simulink model "Main"  (R2025b)
settings: Solver=VariableStepAuto  StartTime=0.0  StopTime=20  RelTol=1e-3
PreLoadFcn:
  | Set_parameters
InitFcn:
  | Set_parameters;
values from neighbouring files (symbols this model uses):
  Date0 = 2460000    [Set_parameters.m]
undefined symbols (not defined in the file or in its folder): Aero, Init, Mass, Prop
libraries: simulink x1
settings Model: Creator=junho  LastModifiedBy=tmej1020

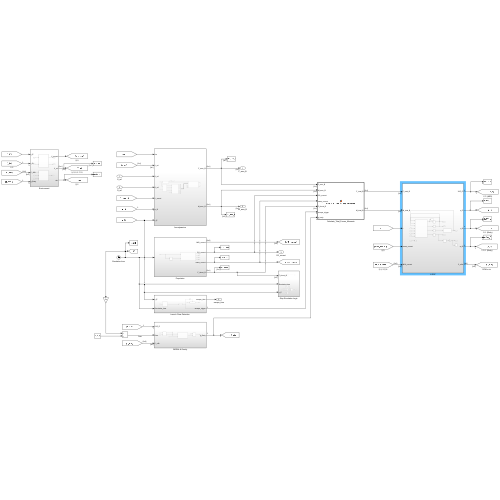
[thumbnail: Simulink's stored preview of the top-level diagram]
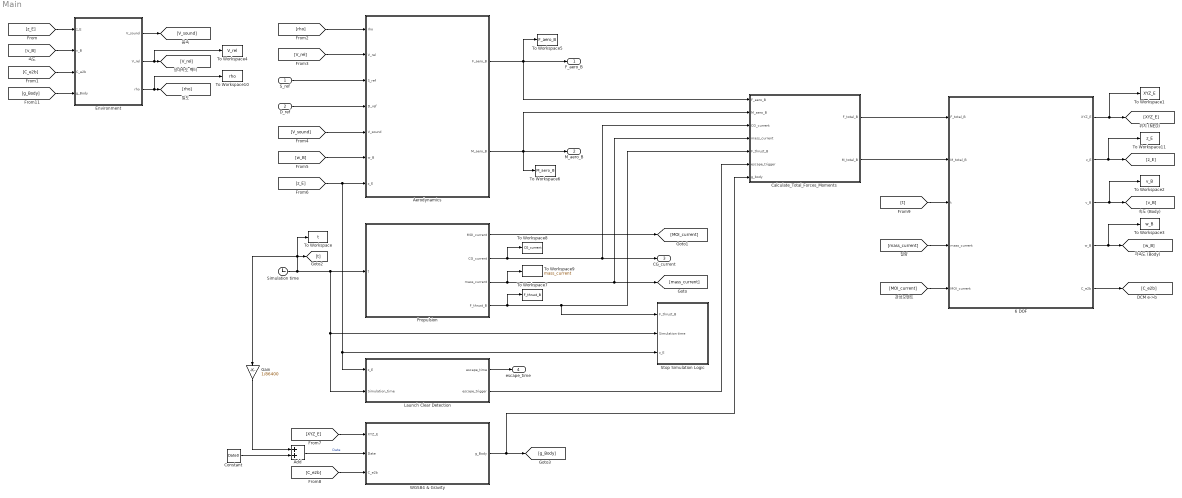
== system Main ==
  S_ref : Inport
  D_ref : Inport  Port=2
  "6 DOF " : Subsystem
  Add : Sum
  Aerodynamics : Subsystem
  Calculate_Total_Forces_Moments : MATLAB Function  TreatAsAtomicUnit=on
  Constant : Constant  Value=Date0
  Environment : Subsystem
  Gain : Gain  Gain=1/86400
  Launch Clear Detection : Subsystem
  Propulsion : Subsystem
  Simulation time : Clock
  Stop Simulation Logic : Subsystem
  To Workspace : ToWorkspace  VariableName=t  SampleTime=-1
  To Workspace1 : ToWorkspace  VariableName=XYZ_E  SampleTime=-1
  To Workspace10 : ToWorkspace  VariableName=rho  SaveFormat=Timeseries  SampleTime=-1
  To Workspace11 : ToWorkspace  VariableName=z_E  SampleTime=-1
  To Workspace2 : ToWorkspace  VariableName=v_B  SaveFormat=Timeseries  SampleTime=-1
  To Workspace3 : ToWorkspace  VariableName=w_B  SaveFormat=Timeseries  SampleTime=-1
  To Workspace4 : ToWorkspace  VariableName=V_rel  SaveFormat=Timeseries  SampleTime=-1
  To Workspace5 : ToWorkspace  VariableName=F_aero_B  SaveFormat=Timeseries  SampleTime=-1
  To Workspace6 : ToWorkspace  VariableName=M_aero_B  SaveFormat=Timeseries  SampleTime=-1
  To Workspace7 : ToWorkspace  VariableName=F_thrust_B  SampleTime=-1
  To Workspace8 : ToWorkspace  VariableName=CG_current  SaveFormat=Timeseries  SampleTime=-1
  To Workspace9 : ToWorkspace  VariableName=mass_current  SaveFormat=Timeseries  SampleTime=-1
  WGS84 & Gravity : Subsystem
  F_aero_B : Outport
  M_aero_B : Outport  Port=2
  CG_current : Outport  Port=3
  escape_time : Outport  Port=4
  wires:
  [XYZ_E] -> WGS84 & Gravity/1(XYZ_E)
  WGS84 & Gravity/1(g_Body) -> [g_Body], Calculate_Total_Forces_Moments/7(g_body)
  Add/1 -> WGS84 & Gravity/2(Date)  "Date"
  [C_e2b] -> WGS84 & Gravity/3(C_e2b)
  [rho] -> Aerodynamics/1(rho)
  [V_rel] -> Aerodynamics/2(V_rel)
  S_ref/1 -> Aerodynamics/3(S_ref)
  D_ref/1 -> Aerodynamics/4(D_ref)
  [V_sound] -> Aerodynamics/5(V_sound)
  [z_E] -> Launch Clear Detection/1(z_E), Stop Simulation Logic/3(z_E), Aerodynamics/7(z_E)
  Aerodynamics/1(F_aero_B) -> F_aero_B/1, Calculate_Total_Forces_Moments/1(F_aero_B), To Workspace5/1
  Aerodynamics/2(M_aero_B) -> M_aero_B/1, To Workspace6/1, Calculate_Total_Forces_Moments/2(M_aero_B)
  [w_B] -> Aerodynamics/6(w_B)
  Simulation time/1 -> Launch Clear Detection/2(Simulation_time), Stop Simulation Logic/2(Simulation time), Propulsion/1(t), To Workspace/1, Gain/1, [t]
  Propulsion/4(F_thrust_B) -> Stop Simulation Logic/1(F_thrust_B), Calculate_Total_Forces_Moments/5(F_thrust_B), To Workspace7/1
  Propulsion/1(MOI_current) -> [MOI_current]
  Propulsion/2(CG_current) -> To Workspace8/1, CG_current/1, Calculate_Total_Forces_Moments/3(CG_current)
  Propulsion/3(mass_current) -> To Workspace9/1, [mass_current], Calculate_Total_Forces_Moments/4(mass_current)
  Launch Clear Detection/1(escape_time) -> escape_time/1
  Launch Clear Detection/2(escape_trigger) -> Calculate_Total_Forces_Moments/6(escape_trigger)
  Calculate_Total_Forces_Moments/2(M_total_B) -> "6 DOF "/2(M_total_B)
  Calculate_Total_Forces_Moments/1(F_total_B) -> "6 DOF "/1(F_total_B)
  "6 DOF "/1(XYZ_E) -> [XYZ_E], To Workspace1/1
  [MOI_current] -> "6 DOF "/5(MOI_current)
  "6 DOF "/4(w_B) -> To Workspace3/1, [w_B]
  "6 DOF "/2(z_E) -> To Workspace11/1, [z_E]
  [mass_current] -> "6 DOF "/4(mass_current)
  "6 DOF "/3(v_B) -> To Workspace2/1, [v_B]
  "6 DOF "/5(C_e2b) -> [C_e2b]
  [v_B] -> Environment/2(v_B)
  Environment/3(rho) -> To Workspace10/1, [rho]
  [C_e2b] -> Environment/3(C_e2b)
  [z_E] -> Environment/1(z_E)
  Environment/2(V_rel) -> To Workspace4/1, [V_rel]
  Environment/1(V_sound) -> [V_sound]
  [t] -> "6 DOF "/3(t)
  Constant/1 -> Add/2
  Gain/1 -> Add/1
  [g_Body] -> Environment/4(g_Body)

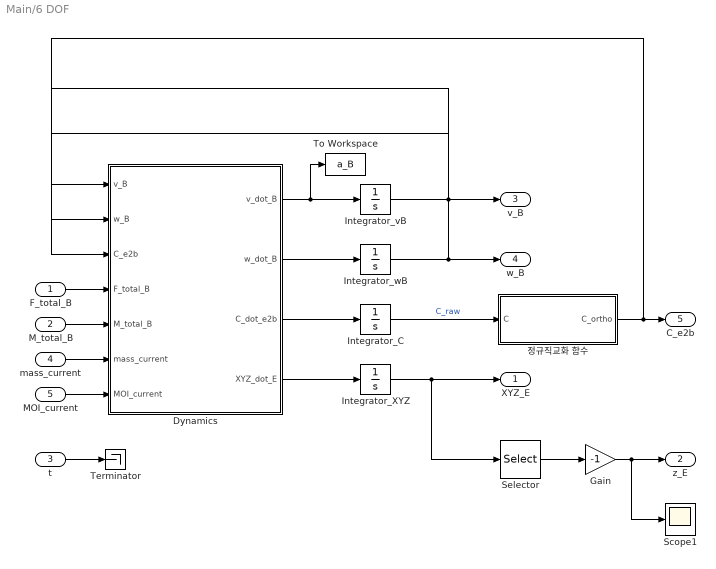
== system Main/6 DOF  ==
  F_total_B : Inport
  M_total_B : Inport  Port=2
  t : Inport  Port=3
  mass_current : Inport  Port=4
  MOI_current : Inport  Port=5
  Dynamics : MATLAB Function  TreatAsAtomicUnit=on
  Gain : Gain  Gain=-1
  Integrator_C : Integrator  InitialCondition=Init.C0_e2b
  Integrator_XYZ : Integrator  InitialCondition=zeros(3,1)
  Integrator_vB : Integrator  InitialCondition=zeros(3,1)
  Integrator_wB : Integrator  InitialCondition=zeros(3,1)
  Scope1 : Scope
      settings: ActiveDisplayYMinimum=-57.51768994793359  ActiveDisplayYMaximum=364.68499660349511
  Selector : Selector  InputPortWidth=3  IndexOptions=Index vector (dialog)  Indices=3  OutputSizes=1
  Terminator : Terminator
  To Workspace : ToWorkspace  VariableName=a_B  SaveFormat=Timeseries  SampleTime=-1
  정규직교화 함수 : MATLAB Function  TreatAsAtomicUnit=on
  XYZ_E : Outport
  z_E : Outport  Port=2
  v_B : Outport  Port=3
  w_B : Outport  Port=4
  C_e2b : Outport  Port=5
  wires:
  Integrator_vB/1 -> v_B/1, Dynamics/1(v_B)
  Integrator_wB/1 -> w_B/1, Dynamics/2(w_B)
  Integrator_XYZ/1 -> Selector/1, XYZ_E/1
  F_total_B/1 -> Dynamics/4(F_total_B)
  M_total_B/1 -> Dynamics/5(M_total_B)
  mass_current/1 -> Dynamics/6(mass_current)
  MOI_current/1 -> Dynamics/7(MOI_current)
  Dynamics/1(v_dot_B) -> To Workspace/1, Integrator_vB/1
  Dynamics/2(w_dot_B) -> Integrator_wB/1
  Dynamics/3(C_dot_e2b) -> Integrator_C/1
  Dynamics/4(XYZ_dot_E) -> Integrator_XYZ/1
  Selector/1 -> Gain/1
  Integrator_C/1 -> 정규직교화 함수/1(C)  "C_raw"
  정규직교화 함수/1(C_ortho) -> Dynamics/3(C_e2b), C_e2b/1
  t/1 -> Terminator/1
  Gain/1 -> Scope1/1, z_E/1

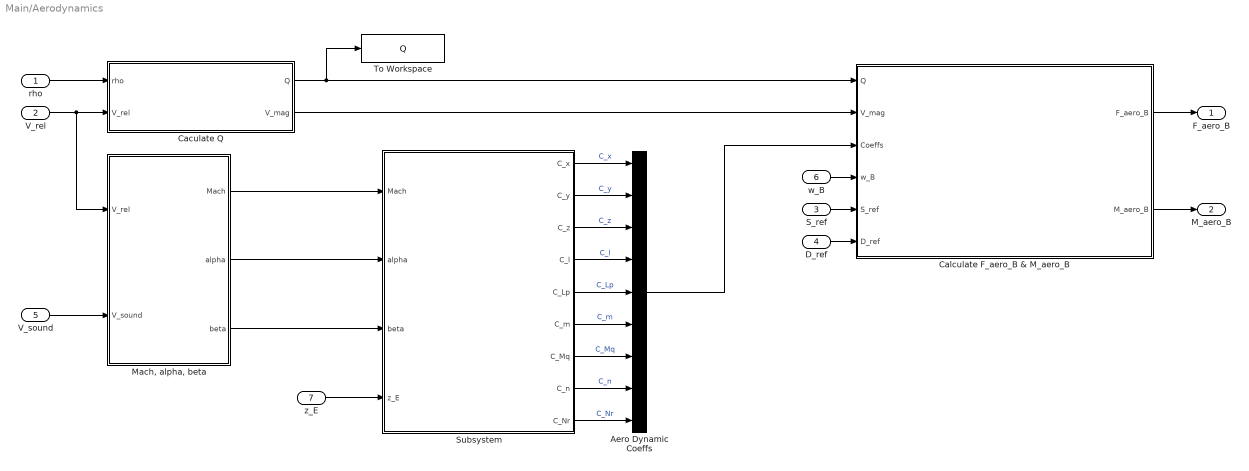
== system Main/Aerodynamics ==
  rho : Inport
  V_rel : Inport  Port=2
  S_ref : Inport  Port=3
  D_ref : Inport  Port=4
  V_sound : Inport  Port=5
  w_B : Inport  Port=6
  z_E : Inport  Port=7
  Aero Dynamic Coeffs : BusCreator  Inputs=9
  Caculate Q : MATLAB Function  TreatAsAtomicUnit=on
  Calculate F_aero_B & M_aero_B : MATLAB Function  TreatAsAtomicUnit=on
  "Mach, alpha, beta " : MATLAB Function  TreatAsAtomicUnit=on
  Subsystem : Subsystem
  To Workspace : ToWorkspace  VariableName=Q  SaveFormat=Timeseries  SampleTime=-1
  F_aero_B : Outport
  M_aero_B : Outport  Port=2
  wires:
  rho/1 -> Caculate Q/1(rho)
  V_rel/1 -> "Mach, alpha, beta "/1(V_rel), Caculate Q/2(V_rel)
  V_sound/1 -> "Mach, alpha, beta "/2(V_sound)
  "Mach, alpha, beta "/1(Mach) -> Subsystem/1(Mach)
  "Mach, alpha, beta "/2(alpha) -> Subsystem/2(alpha)
  "Mach, alpha, beta "/3(beta) -> Subsystem/3(beta)
  z_E/1 -> Subsystem/4(z_E)
  S_ref/1 -> Calculate F_aero_B & M_aero_B/5(S_ref)
  D_ref/1 -> Calculate F_aero_B & M_aero_B/6(D_ref)
  Aero Dynamic Coeffs/1 -> Calculate F_aero_B & M_aero_B/3(Coeffs)
  Calculate F_aero_B & M_aero_B/1(F_aero_B) -> F_aero_B/1
  Calculate F_aero_B & M_aero_B/2(M_aero_B) -> M_aero_B/1
  Subsystem/1(C_x) -> Aero Dynamic Coeffs/1  "C_x"
  Subsystem/2(C_y) -> Aero Dynamic Coeffs/2  "C_y"
  Subsystem/3(C_z) -> Aero Dynamic Coeffs/3  "C_z"
  Subsystem/4(C_l) -> Aero Dynamic Coeffs/4  "C_l"
  Subsystem/5(C_Lp) -> Aero Dynamic Coeffs/5  "C_Lp"
  Subsystem/6(C_m) -> Aero Dynamic Coeffs/6  "C_m"
  Subsystem/7(C_Mq) -> Aero Dynamic Coeffs/7  "C_Mq"
  Subsystem/8(C_n) -> Aero Dynamic Coeffs/8  "C_n"
  Subsystem/9(C_Nr) -> Aero Dynamic Coeffs/9  "C_Nr"
  Caculate Q/1(Q) -> To Workspace/1, Calculate F_aero_B & M_aero_B/1(Q)
  w_B/1 -> Calculate F_aero_B & M_aero_B/4(w_B)
  Caculate Q/2(V_mag) -> Calculate F_aero_B & M_aero_B/2(V_mag)

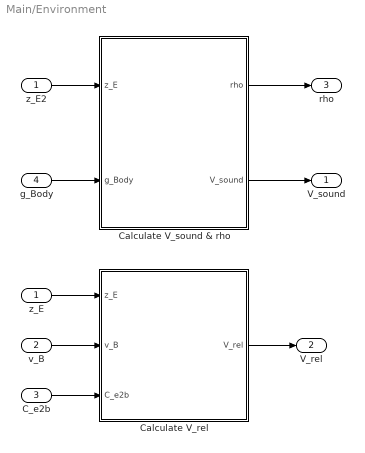
== system Main/Environment ==
  z_E : Inport
  v_B : Inport  Port=2
  C_e2b : Inport  Port=3
  g_Body : Inport  Port=4
  Calculate V_rel : MATLAB Function  TreatAsAtomicUnit=on
  Calculate V_sound & rho : MATLAB Function  TreatAsAtomicUnit=on
  z_E2 : InportShadow
  V_sound : Outport
  V_rel : Outport  Port=2
  rho : Outport  Port=3
  wires:
  z_E/1 -> Calculate V_rel/1(z_E)
  Calculate V_rel/1(V_rel) -> V_rel/1
  z_E2/1 -> Calculate V_sound & rho/1(z_E)
  Calculate V_sound & rho/2(V_sound) -> V_sound/1
  Calculate V_sound & rho/1(rho) -> rho/1
  v_B/1 -> Calculate V_rel/2(v_B)
  C_e2b/1 -> Calculate V_rel/3(C_e2b)
  g_Body/1 -> Calculate V_sound & rho/2(g_Body)

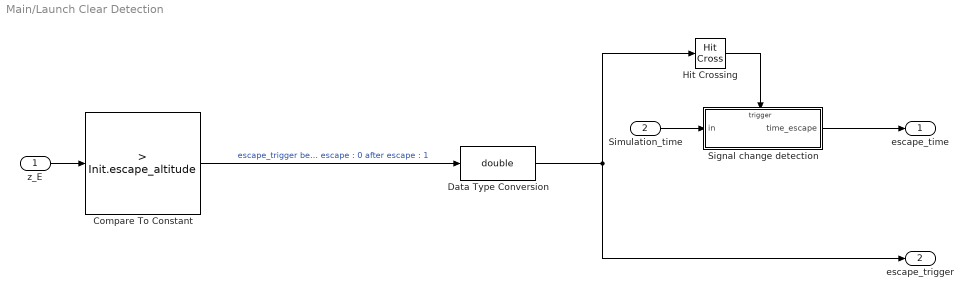
== system Main/Launch Clear Detection ==
  z_E : Inport
  Simulation_time : Inport  Port=2
  Compare To Constant : simulink/Logic and Bit Operations/Compare To Constant  relop=>  const=Init.escape_altitude  OutDataTypeStr=boolean
  Data Type Conversion : DataTypeConversion  OutDataTypeStr=double  SaturateOnIntegerOverflow=off  RndMeth=Floor
  Hit Crossing : HitCross  HitCrossingOffset=0.5  HitCrossingDirection=rising
  "Signal change detection " : Subsystem  TreatAsAtomicUnit=on
  escape_time : Outport
  escape_trigger : Outport  Port=2
  wires:
  z_E/1 -> Compare To Constant/1
  Compare To Constant/1 -> Data Type Conversion/1  "escape_trigger  before escape : 0 after escape : 1"
  Hit Crossing/1 -> "Signal change detection "/Trigger
  "Signal change detection "/1(time_escape) -> escape_time/1
  Data Type Conversion/1 -> escape_trigger/1, Hit Crossing/1
  Simulation_time/1 -> "Signal change detection "/1(in)

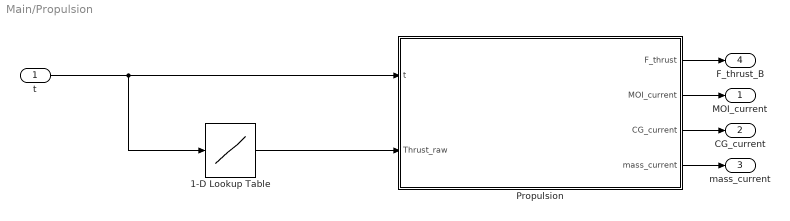
== system Main/Propulsion ==
  t : Inport
  1-D Lookup Table : Lookup_n-D  NumberOfTableDimensions=1  BreakpointsForDimension1=Prop.t_thrust  Table=Prop.F_thrust  ExtrapMethod=Clip  InternalRulePriority=Speed  RndMeth=Simplest
  Propulsion : MATLAB Function  TreatAsAtomicUnit=on
  MOI_current : Outport
  CG_current : Outport  Port=2
  mass_current : Outport  Port=3
  F_thrust_B : Outport  Port=4
  wires:
  t/1 -> 1-D Lookup Table/1, Propulsion/1(t)
  1-D Lookup Table/1 -> Propulsion/2(Thrust_raw)
  Propulsion/4(mass_current) -> mass_current/1
  Propulsion/3(CG_current) -> CG_current/1
  Propulsion/2(MOI_current) -> MOI_current/1
  Propulsion/1(F_thrust) -> F_thrust_B/1

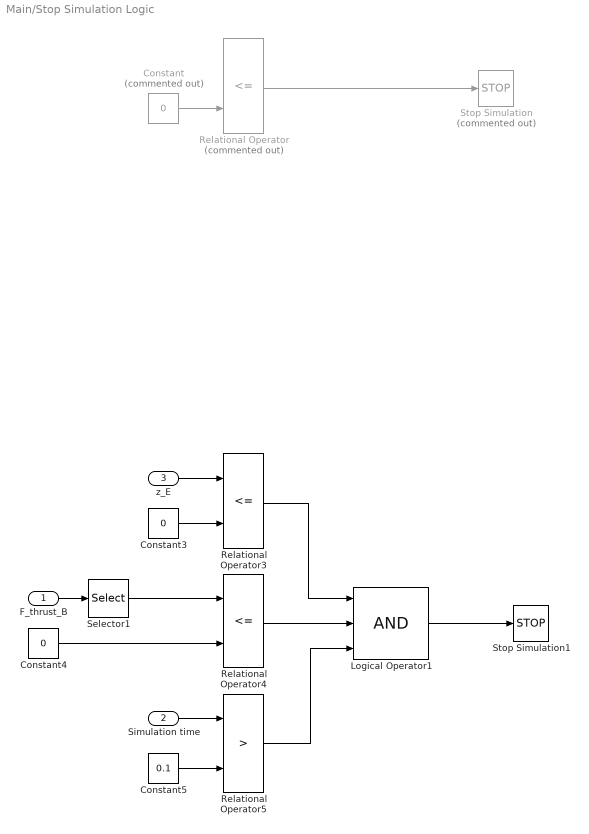
== system Main/Stop Simulation Logic ==
  F_thrust_B : Inport
  Simulation time : Inport  Port=2
  z_E : Inport  Port=3
  Constant : Constant  Commented=on  Value=0
  Constant3 : Constant  Value=0
  Constant4 : Constant  Value=0
  Constant5 : Constant  Value=0.1
  Logical Operator1 : Logic  Inputs=3  AllPortsSameDT=off  OutDataTypeStr=boolean
  Relational Operator : RelationalOperator  Commented=on  Operator=<=  OutDataTypeStr=boolean  RndMeth=Simplest  InputSameDT=off
  Relational Operator3 : RelationalOperator  Operator=<=  OutDataTypeStr=boolean  RndMeth=Simplest  InputSameDT=off
  Relational Operator4 : RelationalOperator  Operator=<=  OutDataTypeStr=boolean  RndMeth=Simplest  InputSameDT=off
  Relational Operator5 : RelationalOperator  Operator=>  OutDataTypeStr=boolean  RndMeth=Simplest  InputSameDT=off
  Selector1 : Selector  InputPortWidth=3  IndexOptions=Index vector (dialog)  Indices=1  OutputSizes=1
  Stop Simulation : Stop  Commented=on
  Stop Simulation1 : Stop
  wires:
  Relational Operator/1 -> Stop Simulation/1
  Constant/1 -> Relational Operator/2
  Selector1/1 -> Relational Operator4/1
  Relational Operator3/1 -> Logical Operator1/1
  Constant5/1 -> Relational Operator5/2
  Constant3/1 -> Relational Operator3/2
  Relational Operator5/1 -> Logical Operator1/3
  Constant4/1 -> Relational Operator4/2
  Relational Operator4/1 -> Logical Operator1/2
  Logical Operator1/1 -> Stop Simulation1/1
  z_E/1 -> Relational Operator3/1
  Simulation time/1 -> Relational Operator5/1
  F_thrust_B/1 -> Selector1/1

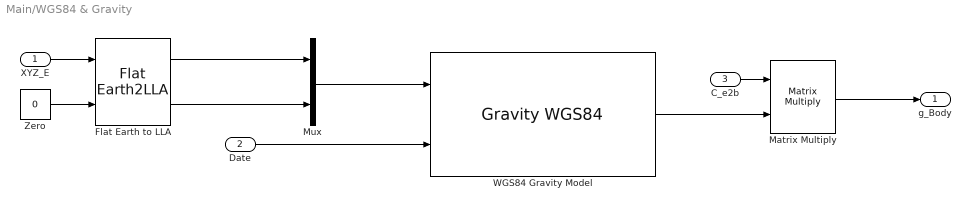
== system Main/WGS84 & Gravity ==
  XYZ_E : Inport
  Date : Inport  Port=2
  C_e2b : Inport  Port=3
  Flat Earth to LLA : FlatEarth2LLA  LL0=[Init.latitude_initial, Init.logitutde_initial]
  Matrix Multiply : Product  Multiplication=Matrix(*)
  Mux : Mux  Inputs=2
  "WGS84 Gravity Model  " : GravityWGS84  model=WGS84 Exact  no_atmos=off  jd_loc=on  month=February  day=19  year=2026  no_centrifugal=off
  Zero : Constant  Value=0  OutDataTypeStr=Inherit: Inherit via back propagation
  g_Body : Outport
  wires:
  XYZ_E/1 -> Flat Earth to LLA/1
  Date/1 -> "WGS84 Gravity Model  "/2
  Zero/1 -> Flat Earth to LLA/2
  Flat Earth to LLA/1 -> Mux/1
  Flat Earth to LLA/2 -> Mux/2
  Mux/1 -> "WGS84 Gravity Model  "/1
  "WGS84 Gravity Model  "/1 -> Matrix Multiply/2
  C_e2b/1 -> Matrix Multiply/1
  Matrix Multiply/1 -> g_Body/1

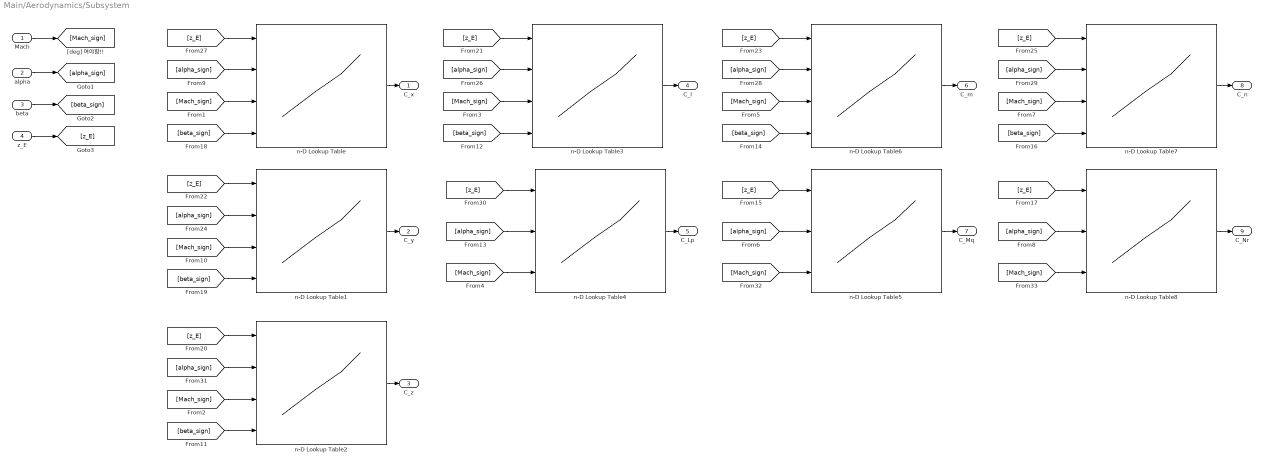
== system Main/Aerodynamics/Subsystem ==
  Mach : Inport
  alpha : Inport  Port=2
  beta : Inport  Port=3
  z_E : Inport  Port=4
  n-D Lookup Table : Lookup_n-D  NumberOfTableDimensions=4  BreakpointsForDimension1=Aero.altVec  BreakpointsForDimension2=Aero.alphaVec  BreakpointsForDimension3=Aero.machVec  BreakpointsForDimension4=Aero.betaVec  Table=Aero.CA_DB  InternalRulePriority=Speed  RndMeth=Simplest
      settings: InputPortMap=u0,u1,u2,u3
  n-D Lookup Table1 : Lookup_n-D  NumberOfTableDimensions=4  BreakpointsForDimension1=Aero.altVec  BreakpointsForDimension2=Aero.alphaVec  BreakpointsForDimension3=Aero.machVec  BreakpointsForDimension4=Aero.betaVec  Table=Aero.CY_DB  InternalRulePriority=Speed  RndMeth=Simplest
      settings: InputPortMap=u0,u1,u2,u3
  n-D Lookup Table2 : Lookup_n-D  NumberOfTableDimensions=4  BreakpointsForDimension1=Aero.altVec  BreakpointsForDimension2=Aero.alphaVec  BreakpointsForDimension3=Aero.machVec  BreakpointsForDimension4=Aero.betaVec  Table=Aero.CN_DB  InternalRulePriority=Speed  RndMeth=Simplest
      settings: InputPortMap=u0,u1,u2,u3
  n-D Lookup Table3 : Lookup_n-D  NumberOfTableDimensions=4  BreakpointsForDimension1=Aero.altVec  BreakpointsForDimension2=Aero.alphaVec  BreakpointsForDimension3=Aero.machVec  BreakpointsForDimension4=Aero.betaVec  Table=Aero.CLL_DB  InternalRulePriority=Speed  RndMeth=Simplest
      settings: InputPortMap=u0,u1,u2,u3
  n-D Lookup Table4 : Lookup_n-D  NumberOfTableDimensions=3  BreakpointsForDimension1=Aero.altVec_dynamic  BreakpointsForDimension2=Aero.alphaVec  BreakpointsForDimension3=Aero.machVec  Table=Aero.CLLP_DB  InternalRulePriority=Speed  RndMeth=Simplest
      settings: InputPortMap=u0,u1,u2
  n-D Lookup Table5 : Lookup_n-D  NumberOfTableDimensions=3  BreakpointsForDimension1=Aero.altVec_dynamic  BreakpointsForDimension2=Aero.alphaVec  BreakpointsForDimension3=Aero.machVec  Table=Aero.CMQ_DB  InternalRulePriority=Speed  RndMeth=Simplest
      settings: InputPortMap=u0,u1,u2
  n-D Lookup Table6 : Lookup_n-D  NumberOfTableDimensions=4  BreakpointsForDimension1=Aero.altVec  BreakpointsForDimension2=Aero.alphaVec  BreakpointsForDimension3=Aero.machVec  BreakpointsForDimension4=Aero.betaVec  Table=Aero.CM_DB  InternalRulePriority=Speed  RndMeth=Simplest
      settings: InputPortMap=u0,u1,u2,u3
  n-D Lookup Table7 : Lookup_n-D  NumberOfTableDimensions=4  BreakpointsForDimension1=Aero.altVec  BreakpointsForDimension2=Aero.alphaVec  BreakpointsForDimension3=Aero.machVec  BreakpointsForDimension4=Aero.betaVec  Table=Aero.CLN_DB  InternalRulePriority=Speed  RndMeth=Simplest
      settings: InputPortMap=u0,u1,u2,u3
  n-D Lookup Table8 : Lookup_n-D  NumberOfTableDimensions=3  BreakpointsForDimension1=Aero.altVec_dynamic  BreakpointsForDimension2=Aero.alphaVec  BreakpointsForDimension3=Aero.machVec  Table=Aero.CLNR_DB  InternalRulePriority=Speed  RndMeth=Simplest
      settings: InputPortMap=u0,u1,u2
  C_x : Outport
  C_y : Outport  Port=2
  C_z : Outport  Port=3
  C_l : Outport  Port=4
  C_Lp : Outport  Port=5
  C_m : Outport  Port=6
  C_Mq : Outport  Port=7
  C_n : Outport  Port=8
  C_Nr : Outport  Port=9
  wires:
  Mach/1 -> [Mach_sign]
  alpha/1 -> [alpha_sign]
  beta/1 -> [beta_sign]
  z_E/1 -> [z_E]
  n-D Lookup Table/1 -> C_x/1
  n-D Lookup Table1/1 -> C_y/1
  n-D Lookup Table2/1 -> C_z/1
  n-D Lookup Table3/1 -> C_l/1
  n-D Lookup Table4/1 -> C_Lp/1
  n-D Lookup Table6/1 -> C_m/1
  n-D Lookup Table5/1 -> C_Mq/1
  n-D Lookup Table7/1 -> C_n/1
  n-D Lookup Table8/1 -> C_Nr/1
  [alpha_sign] -> n-D Lookup Table4/2
  [z_E] -> n-D Lookup Table/1
  [alpha_sign] -> n-D Lookup Table/2
  [Mach_sign] -> n-D Lookup Table/3
  [beta_sign] -> n-D Lookup Table/4
  [alpha_sign] -> n-D Lookup Table1/2
  [Mach_sign] -> n-D Lookup Table1/3
  [z_E] -> n-D Lookup Table1/1
  [beta_sign] -> n-D Lookup Table1/4
  [alpha_sign] -> n-D Lookup Table3/2
  [Mach_sign] -> n-D Lookup Table3/3
  [z_E] -> n-D Lookup Table3/1
  [beta_sign] -> n-D Lookup Table3/4
  [alpha_sign] -> n-D Lookup Table6/2
  [Mach_sign] -> n-D Lookup Table6/3
  [z_E] -> n-D Lookup Table6/1
  [beta_sign] -> n-D Lookup Table6/4
  [alpha_sign] -> n-D Lookup Table7/2
  [Mach_sign] -> n-D Lookup Table7/3
  [z_E] -> n-D Lookup Table7/1
  [beta_sign] -> n-D Lookup Table7/4
  [alpha_sign] -> n-D Lookup Table2/2
  [Mach_sign] -> n-D Lookup Table2/3
  [z_E] -> n-D Lookup Table2/1
  [beta_sign] -> n-D Lookup Table2/4
  [z_E] -> n-D Lookup Table4/1
  [Mach_sign] -> n-D Lookup Table4/3
  [z_E] -> n-D Lookup Table5/1
  [alpha_sign] -> n-D Lookup Table5/2
  [Mach_sign] -> n-D Lookup Table5/3
  [z_E] -> n-D Lookup Table8/1
  [alpha_sign] -> n-D Lookup Table8/2
  [Mach_sign] -> n-D Lookup Table8/3

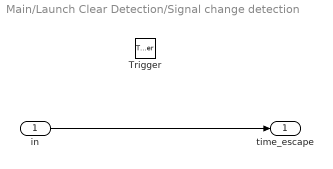
== system Main/Launch Clear Detection/Signal change detection  ==
  in : Inport
  Trigger : TriggerPort  VariantControl=(inherit)
  time_escape : Outport
  wires:
  in/1 -> time_escape/1

== matlab function Main/Environment/Calculate V_sound & rho ==
  data: rho output; z_E input; V_sound output; g_Body input
function [rho, V_sound] = Calculate_V_sound_and_rho(z_E, g_Body)

%% 입력: z_E [m] 
%% 출력: rho [kg/m^3], V_sound [m/s]

%% 상수값 정의 국제표준대기 참고
T0    = 288.15;     % [K]
p0    = 101325.0;   % [Pa]
%g0    = 9.80665;    % [m/s^2]
g = norm(g_Body);
R     = 287.05;     % [J/(kg·K)]
k     = 1.4;        % [-]
L     = 0.0065;     % [K/m] lapse rate (0~11 km)

%% 고도 상한, 하한선 설정 (대류권 구간)
if z_E < 0
    z_E = 0;
elseif z_E > 11000
    z_E = 11000;
end

%% 대류권 내 계산 모델 
T = T0 - L*z_E;                   % 온도 [K]
p = p0 * (T/T0)^(g/(R*L));       % 압력 [Pa]

%% 출력
rho = p/(R*T);                % 밀도 [kg/m^3]
V_sound = sqrt(k*R*T);        % 음속 [m/s]
end

== matlab function Main/Aerodynamics/Mach, alpha, beta  ==
  data: V_rel input; Mach output; V_sound input; alpha output; beta output
function [Mach, alpha, beta] = Mach_alpha_beta(V_rel, V_sound)
    % 입력: V_rel [u_rel; v_rel; w_rel], V_sound (음속)
    
    u_rel = V_rel(1);
    v_rel = V_rel(2);
    w_rel = V_rel(3);
    
    V_mag = sqrt(u_rel^2 + v_rel^2 + w_rel^2);
    
    % --- 예외 처리 시작 ---
    eps_v = 1e-6; % 속도 임계값 (m/s)
    
    if V_mag < eps_v
        % 속도가 거의 0인 경우 (정지 상태 등)
        Mach = 0;
        alpha = 0;
        beta = 0;
    else
        % 일반적인 비행 상태
        Mach = V_mag / V_sound;
        
        % rad2deg 함수를 사용하여 라디안을 디그리로 변환
        alpha_rad = atan2(w_rel, u_rel);
        alpha = rad2deg(alpha_rad); 
        
        beta_rad = asin(max(min(v_rel / V_mag, 1), -1));
        beta = rad2deg(beta_rad);
    end
    % --- 예외 처리 끝 ---
end

== matlab function Main/Aerodynamics/Caculate Q ==
  data: rho input; Q output; V_rel input; V_mag output
function [Q,V_mag] = Calculate_Q(rho, V_rel)
    % 이 함수는 공기 밀도(rho)와 상대 속도 벡터(V_rel)를 받아 동압(Q)을 계산합니다.
    % V_rel: [u; v; w] 형태의 3x1 벡터라고 가정합니다.
    
    % 1. 속도 벡터의 크기(Magnitude) 계산
    % V_rel이 스칼라(TAS)라면 단순히 V_mag = V_rel; 로 작성해도 됩니다.
    V_mag = norm(V_rel); 
    
    % 2. 동압 공식 적용: Q = 0.5 * rho * V^2
    Q = 0.5 * rho * V_mag^2;
end

== matlab function Main/Aerodynamics/Calculate F_aero_B & M_aero_B ==
  data: Q input; V_mag input; Coeffs input Bus: AeroCoeffBus; w_B input; S_ref input; D_ref input; F_aero_B output; M_aero_B output
function [F_aero_B, M_aero_B] = Calculate_F_aero_B_and_M_aero_B(Q, V_mag, Coeffs, w_B, S_ref, D_ref)
    % 입력 정의:
    % Q       : 동압 (Dynamic Pressure) [N/m^2]
    % V_mag   : 속도 크기 (Velocity Magnitude) [m/s]
    % w_B     : 각속도 벡터 [p; q; r] [rad/s]
    % Coeffs  : Bus Creator로부터 온 9개 공력 계수 구조체 (C_x, C_y, C_z, C_l, C_m, C_n, C_Lp, C_Mq, C_Nr)
    % S_ref   : 기준 면적 (Reference Area) [m^2]
    % D_ref   : 기준 직경 (Reference Diameter) [m]

    % 출력 정의:
    % F_aero_B : 기체 좌표계 공력 힘 [Fx; Fy; Fz] [N]
    % M_aero_B : 기체 좌표계 공력 모멘트 [Ml; Mm; Mn] [N*m]
    
    %% 출력 크기 명시
    F_aero_B = zeros(3,1);
    M_aero_B = zeros(3,1);

    %% 1. 각속도 성분 추출 [rad/s]
    p = w_B(1);
    q = w_B(2);
    r = w_B(3);

    %% 2. 수치적 안정성을 위한 속도 임계값 설정
    % 속도가 0인 초기 상태에서 분모가 0이 되어 NaN이 발생하는 것 방지
    eps_v = 1e-6;
    if V_mag < eps_v
        v_denom = eps_v; 
    else
        v_denom = V_mag;
    end

    %% 3. 공력 힘(Aerodynamic Forces) 계산
    % 수식: F = Q * S_ref * [C_x; C_y; C_z]
    F_x = Q * S_ref * Coeffs.C_x;
    F_y = Q * S_ref * Coeffs.C_y;
    F_z = Q * S_ref * Coeffs.C_z;

    F_aero_B = [F_x; F_y; F_z];

    %% 4. 공력 모멘트(Aerodynamic Moments) 계산
    % 수식: M = Q * S_ref * D_ref * [C_l + (D/2v)*C_Lp*p; C_m + (D/2v)*C_Mq*q; C_n + (D/2v)*C_Nr*r]
    
    % 댐핑 팩터 (D/2v) 계산
    damping_factor = D_ref / (2 * v_denom);

    M_l = Q * S_ref * D_ref * (Coeffs.C_l + damping_factor * Coeffs.C_Lp * p);
    M_m = Q * S_ref * D_ref * (Coeffs.C_m + damping_factor * Coeffs.C_Mq * q);
    M_n = Q * S_ref * D_ref * (Coeffs.C_n + damping_factor * Coeffs.C_Nr * r);

    M_aero_B = [M_l; M_m; M_n];

end

== matlab function Main/Propulsion/Propulsion ==
  data: t input; F_thrust output; Thrust_raw input; MOI_current output; CG_current output; mass_current output; Mass parameter; Prop parameter
function [F_thrust, MOI_current, CG_current, mass_current] = Propulsion(t, Thrust_raw, Mass, Prop)
    % 입력:
    % t          : 시뮬레이션 시간 [s] (Clock 블록)
    % Thrust_raw : Lookup Table에서 온 추력 값 [N]
    % Mass       : 질량/관성 구조체 (Mass.mass_initial 등)
    % Prop       : 추진 구조체 (Prop.m_dot_negative 등)

    t_burn = Prop.burn_time;

    if t <= t_burn
        % 1. 연소 중: 1차 함수 모델링 (상수 기울기 적용)
        mass_current = Mass.mass_initial - Prop.mass_dot_negative * t;
        MOI_current  = Mass.MOI_initial - Prop.MOI_dot_negative * t;
        CG_current   = Prop.CG_initial - Prop.CG_dot_negative * t;
        F_thrust     = [Thrust_raw;0;0];
    else
        % 2. 연소 종료 후: 최종 값으로 고정
        mass_current = Mass.mass_final;
        MOI_current  = Mass.MOI_final;
        CG_current   = Prop.CG_final;
        F_thrust     = [0;0;0];
    end
end

== matlab function Main/Calculate_Total_Forces_Moments ==
  data: F_aero_B input; M_aero_B input; CG_current input; mass_current input; F_thrust_B input; escape_trigger input; g_body input; F_total_B output; M_total_B output
%{
function [F_total_B,M_total_B] = Calculate_Total_Forces_Moments(F_aero_B, M_aero_B, CG_current, mass_current, F_thrust, escape_trigger, g_body)
    % 입력 정의:
    % F_aero_B      : [Fx; Fy; Fz] 공력 [N]
    % M_aero_B      : [Ml; Mm; Mn] 공력 모멘트 [N*m]
    % F_thrust_B    : [Thrust_raw; 0; 0] 추력 벡터 [N]
    % mass_current  : 현재 질량 [kg]
    % CG_current    : 노즈로부터 현재 무게중심까지의 거리 [m]
    % escape_trigger: 발사대 이탈 여부 (0: 레일 위, 1: 자유비행)
    % r_MRP         : 초기 무게중심 위치 (Nose 기준 거리) [m] (Parameter)
    % g_body        : 기체좌표계로 변환된 중력가속도 벡터 [m/s^2]
    r_MRP = 1.2;
    %% 1. 중력 벡터 계산 (Body Frame)
    % 입력받은 g_body를 질량과 곱하여 중력 산출
    F_weight_B = mass_current * g_body;

    %% 2. 총 외력 합산 (Total Force)
    
    F_total_B = F_thrust + F_aero_B + F_weight_B;

    %% 3. 총 모멘트 합산 (Total Moment)
    % M_total_B = M_aero_B + (r_MRP - r_BG) x F_aero_B
    % 노즈로부터의 거리 차이를 X축 벡터로 변환
    
    dist_offset = r_MRP - CG_current;
    r_offset_vec = [dist_offset; 0; 0];
    
    % 외적(Cross Product)을 통한 모멘트 보정항 계산
    M_offset_B = cross(r_offset_vec, F_aero_B);
    
    M_total_B = M_aero_B + M_offset_B;

    %% 4. 발사대 구속 로직 (Launch Rail Constraint)
    % escape_trigger가 0(레일 위)일 경우:
    % - 로켓은 X축 방향으로만 움직일 수 있음 (Y, Z 힘 제거)
    % - 로켓은 회전할 수 없음 (모든 모멘트 제거)
    if escape_trigger == 0
        F_total_B(2:3) = 0; % Fy, Fz 제거
        M_total_B(:)   = 0; % Ml, Mm, Mn 제거
    end
end
%}

function [F_total_B,M_total_B] = Calculate_Total_Forces_Moments(F_aero_B, M_aero_B, CG_current, mass_current, F_thrust_B, escape_trigger, g_body)

    % 입력 정의:
    % F_aero_B      : [Fx; Fy; Fz] 공력 [N]
    % M_aero_B      : [Ml; Mm; Mn] 공력 모멘트 [N*m]
    % F_thrust      : 스칼라 추력 또는 [Thrust;0;0] 벡터 [N]
    % mass_current  : 현재 질량 [kg]
    % CG_current    : 노즈로부터 현재 무게중심까지의 거리 [m]
    % escape_trigger: 발사대 이탈 여부 (0: 레일 위, 1: 자유비행)
    % g_body        : 기체좌표계 중력가속도 벡터 [m/s^2]

    %% 출력 크기 미리 지정
    F_total_B = zeros(3,1);
    M_total_B = zeros(3,1);

    %% 기준점(MRP) 위치 [m]
    r_MRP = 1.2;

    %% 입력 형상 강제
    F_aero_B = reshape(F_aero_B, [3,1]);
    M_aero_B = reshape(M_aero_B, [3,1]);
    g_body   = reshape(g_body,   [3,1]);

    % 추력은 스칼라일 수도 있으므로 처리
    if isscalar(F_thrust_B)
        F_thrust_B = [F_thrust_B; 0; 0];
    else
        F_thrust_B = reshape(F_thrust_B, [3,1]);
    end

    %% 1. 중력 벡터 계산 (Body Frame)
    F_weight_B = mass_current * g_body;

    %% 2. 총 외력 합산
    F_total_B = F_thrust_B + F_aero_B + F_weight_B;

    %% 3. 총 모멘트 합산
    % M_total_B = M_aero_B + (r_MRP - CG_current) x F_aero_B

    dist_offset = r_MRP - CG_current;
    r_offset_vec = [dist_offset; 0; 0];
    r_offset_vec = reshape(r_offset_vec, [3,1]);

    M_offset_B = cross(r_offset_vec, F_aero_B);
    M_total_B = M_aero_B + M_offset_B;

    %% 4. 발사대 구속 로직
    if escape_trigger == 0
        F_total_B(2:3) = 0;
        M_total_B(:)   = 0;
    end
end

== matlab function Main/6 DOF /Dynamics ==
  data: v_dot_B output; w_dot_B output; C_dot_e2b output; v_B input; w_B input; C_e2b input; F_total_B input; M_total_B input; mass_current input; MOI_current input; XYZ_dot_E output
function [v_dot_B, w_dot_B, C_dot_e2b, XYZ_dot_E] = Dynamics(v_B, w_B, C_e2b, F_total_B, M_total_B, mass_current, MOI_current)

    %% 출력 크기 명시
    v_dot_B   = zeros(3,1);
    w_dot_B   = zeros(3,1);
    C_dot_e2b = zeros(3,3);

    %% 입력 형상 강제
    v_B       = reshape(v_B,       [3,1]);
    w_B       = reshape(w_B,       [3,1]);
    F_total_B = reshape(F_total_B, [3,1]);
    M_total_B = reshape(M_total_B, [3,1]);
    C_e2b     = reshape(C_e2b,     [3,3]);

    %% 관성모멘트 행렬 형상 정리
    if isequal(size(MOI_current), [3 3])
        I = MOI_current;
    elseif numel(MOI_current) == 9
        I = reshape(MOI_current, [3,3]);
    else
        error('MOI_current must be 3x3 or 9 elements.');
    end

    %% 병진 운동
    v_dot_B = F_total_B / mass_current - cross(w_B, v_B);

    %% 회전 운동
    H = I * w_B;
    w_dot_B = I \ (M_total_B - cross(w_B, H));

    %% 자세행렬 미분
    wx = w_B(1);
    wy = w_B(2);
    wz = w_B(3);

    omega = [  0   -wz   wy;
              wz    0   -wx;
             -wy   wx    0 ];

    C_dot_e2b = omega * C_e2b;

    %% 자세 미분
    XYZ_dot_E = C_e2b.' * v_B;

end

%{
function [v_dot_B, w_dot_B, C_dot_e2b] = Dynamics(v_B, w_B, C_e2b, F_total_B, M_total_B, mass_current, MOI_current)

%% 입력
% v_B        [3x1] 바디 좌표계 속도
% w_B        [3x1] 바디 좌표계 각속도 (p q r)
% C_e2b      [3x3] DCM_earth_to_body
% F_total_B  [3x1] 바디 좌표계 합력
% M_total_B  [3x1] 바디 좌표계 합모멘트
% mass_current  [1x1] 현재 질량
% MOI_current  [3x3] 현재 관성모멘트

%% 출력
% v_dot_B    [3x1] 바디 좌표계 선가속도
% w_dot_B    [3x1] 바디 좌표계 각가속도
% C_dot_e2b  [3x3] DCM_earth_to_body 미분

%% 형상 정리(행/열 혼선 방지) -> 열벡터로 정리
v_B       = v_B(:);
w_B       = w_B(:);
F_total_B = F_total_B(:);
M_total_B = M_total_B(:);

%% 병진 운동 방정식 
% SumF = m*(v_dot_B + w x v)  ->  v_dot = (1/m)*SumF - (w x v)
v_dot_B = F_total_B./mass_current - cross(w_B, v_B);

%% 관성 입력 처리 -> 혹시 몰라서
if numel(MOI_current) == 3            % [Ixx; Iyy; Izz]와 같이 주관성모멘트만 들어왔을 경우
    I = diag(MOI_current(:));         % 대각 관성행렬로 바꿈
else                            
    I = MOI_current;                  % 3×3 관성행렬일 경우 그대로 출력
end

%% 회전 운동 방정식 
% SumM = I*w_dot_B + w x (I*w)  ->  w_dot = I^(-1)*(SumM - w x (I*w))
H = I * w_B;                                  % 각운동량
w_dot_B = I \ (M_total_B - cross(w_B, H));    % 역행렬 대신 \ 사용 (좌측 행렬 나눗셈)

%% DCM 
% C_dot_e2b = omega * C_e2b -> 원동민 선배님 ppt 29p
wx = w_B(1); 
wy = w_B(2); 
wz = w_B(3);
omega = [  0   -wz   wy;
          wz    0   -wx;
         -wy   wx    0 ];    

C_dot_e2b = omega * C_e2b;          % 각속도 벡터를 행렬로 변환해서 행렬곱 실행

end
%}

== matlab function Main/6 DOF /정규직교화 함수 ==
  data: C input; C_ortho output
function C_ortho = Orthonormalize_DCM(C)

c1 = C(:,1);
c2 = C(:,2);

c1 = c1 / max(norm(c1), 1e-12);

c2 = c2 - c1 * (c1.' * c2);
c2 = c2 / max(norm(c2), 1e-12);

c3 = cross(c1, c2);
c3 = c3 / max(norm(c3), 1e-12);

C_ortho = [c1 c2 c3];

== matlab function Main/Environment/Calculate V_rel ==
  data: z_E input; V_rel output; v_B input; C_e2b input
function V_rel  = Calculate_V_rel( z_E, v_B, C_e2b)

%% 입력
% z_E   : 고도 [m] 
% v_B   : 바디 속도 [m/s], 3x1
% C_e2b : DCM (Earth -> Body), 3x3

%% 출력
% V_rel : 바디좌표계에서의 상대속도 [m/s], 벡터값 3x1

%% 1) 무풍 모델 (일단은 무풍 추후에 u, v 데이터값 추가)
u = 0;  v = 0;  w = 0;
wind_E = [u; v; w];          % 지면 좌표계 풍속(3x1)
wind_B = C_e2b * wind_E;     % 바디 좌표계 풍속(3x1)

%% 바람 모델 -> 추후 u, v 추가

% u = interp1(alt, wind_u, z_E, 'linear', 'extrap');
% v = interp1(alt, wind_v, z_E, 'linear', 'extrap');
% w = 0; 
% vq = interp1(x, v, xq)
% x: 이미 알고 있는 데이터의 위치 (x축 값)
% v: 이미 알고 있는 데이터의 실제 값 (y축 값)
% xq: 내가 궁금한, 값을 알고 싶은 새로운 위치 
% vq: 함수가 계산해서 알려주는 추측된 값 
% u, v는 추후 베이스 파라미터에 엑셀표로 삽입

%% 출력
V_rel = v_B - wind_B;        % 상대 속도 벡터 (Body) 3x1
end
